simulink model "TorqueVectoringAlgorithm"  (R2020a)
settings: Solver=VariableStepAuto  StartTime=0.0  StopTime=10.0  RelTol=1e-3  EnableMultiTasking=on
libraries: TorqueVectoringAlgorithmLib x1
settings Model: Creator=Harjot  LastModifiedBy=Harjot
settings OptimizationCC: LifeSpan=inf
settings DebuggingCC: SFUnexpectedBacktrackingDiag=warning  SFNoUnconditionalDefaultTransitionDiag=warning  SFExecutionAtInitializationDiag=none  ArithmeticOperatorsInVariantConditions=warning
settings SFSimCC: SimUseLocalCustomCode=off  CustomCodeUndefinedFunction=UseInterfaceOnly
settings RTWCC: RTWUseLocalCustomCode=off
settings CodeAppCC: StateflowObjectComments=on
settings GRTTargetCC: TargetLangStandard=C89/C90 (ANSI)
settings ConfigComp: CovMetricSettings=dw  CovHtmlReporting=on  CovSaveCumulativeToWorkspaceVar=on  CovSaveSingleToWorkspaceVar=on  CovExternalEMLEnable=off

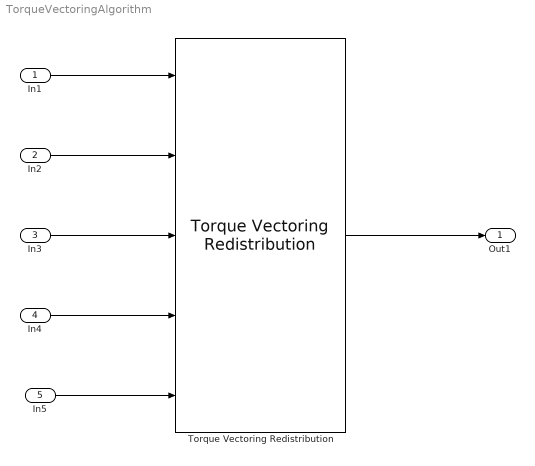
== system TorqueVectoringAlgorithm ==
  In1 : Inport
  In2 : Inport  Port=2
  In3 : Inport  Port=3
  In4 : Inport  Port=4
  In5 : Inport  Port=5
  Torque Vectoring Redistribution : TorqueVectoringAlgorithmLib/Torque Vectoring Redistribution  wheel_1=Front  wheel_2=Left
  Out1 : Outport  VectorParamsAs1DForOutWhenUnconnected=off
  wires:
  In1/1 -> Torque Vectoring Redistribution/1
  In2/1 -> Torque Vectoring Redistribution/2
  In3/1 -> Torque Vectoring Redistribution/3
  In4/1 -> Torque Vectoring Redistribution/4
  In5/1 -> Torque Vectoring Redistribution/5
  Torque Vectoring Redistribution/1 -> Out1/1
